simulink library "MOST_Lib"  (R2020b)
settings: Solver=VariableStepAuto  StartTime=0.0  StopTime=10.0  RelTol=1e-3
undefined symbols (not defined in the file): simu, wind, windTurbine, windturbine, X, Y, Z
libraries: nesl_utility x54, sm_lib x50, simulink x4, simulink_extras x1, pid_lib x1, WECSim_Lib_Body_Elements x1
(part 1 of 3)
settings Model: Creator=d060241  LastModifiedBy=akeeste
settings DebuggingCC: UnconnectedInputMsg=none  UnconnectedOutputMsg=none  UnconnectedLineMsg=none
settings ModelReferenceCC: EnableRefExpFcnMdlSchedulingChecks=off

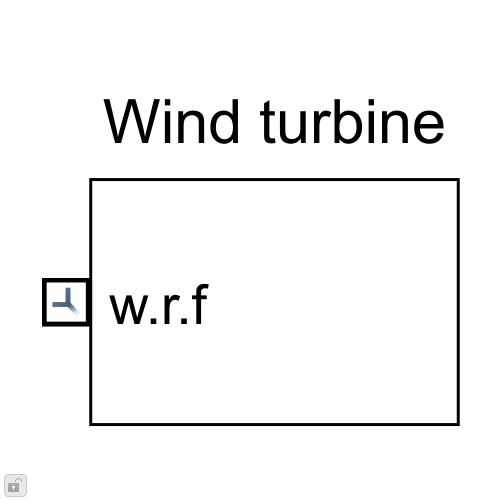
[thumbnail: Simulink's stored preview of the top-level diagram]
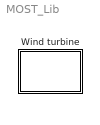
== system MOST_Lib ==
  Wind turbine : Subsystem  VariantControl=sv_1_IEA15MW  mask{windTurbine=windTurbine, BEMstruct=windTurbine.BEMstruct}
      mask prompts: windTurbine "Wind Number:"; BEMstruct "BEM structure"
      mask init:
      | %% Variand sybsystems
      | h = [gcb '/Aerodynamics + Control/Aeroloads/Look-up Tables'];
      | responseName = ['sv_t' num2str(windTurbine.number) '_AeroLoads0'];
      | set_param(h,'VariantControl',responseName);
      | 
      | h = [gcb '/Aerodynamics + Control/Aeroloads/BEM'];
      | responseName = ['sv_t' num2str(windTurbine.number) '_AeroLoads1'];
      | set_param(h,'VariantControl',responseName);
      | 
      | h = [gcb '/Aerodynamics + Control/Control/Baseline'];
      | responseName = ['sv_t' num2str(windTurbine.number) '_control0'];
      | set_param(h,'VariantControl',responseName);
      | 
      | h = [gcb '/Aerodynamics + Control/Control/ROSCO'];
      | responseName = ['sv_t' num2str(windTurbine.number) '_control1'];
      | set_param(h,'VariantControl',responseName);
      | 
      | %% Body properties
      | h1=[gcb '/Tower/Body Properties Tower'];
      | geomFile=windTurbine.geometryFileTower;
      | set_param(h1,'ExtGeomFileName',geomFile);
      | geomType='STEP';
      | 
      | h1=[gcb '/Nacelle/Body Properties Nacelle'];
      | geomFile=windTurbine.geometryFileNacelle;
      | set_param(h1,'ExtGeomFileName',geomFile);
      | geomType='STEP';
      | 
      | h1=[gcb '/Hub/Body Properties Hub'];
      | geomFile=windTurbine.geometryFileHub;
      | set_param(h1,'ExtGeomFileName',geomFile);
      | geomType='STEP';
      | 
      | h1=[gcb '/Blade 1/Blade/Body Properties Blade'];
      | geomFile=windTurbine.geometryFileBlade;
      | set_param(h1,'ExtGeomFileName',geomFile);
      | geomType='STEP';
      | 
      | h1=[gcb '/Blade 2/Blade/Body Properties Blade'];
      | geomFile=windTurbine.geometryFileBlade;
      | set_param(h1,'ExtGeomFileName',geomFile);
      | geomType='STEP';
      | 
      | h1=[gcb '/Blade 3/Blade/Body Properties Blade'];
      | geomFile=windTurbine.geometryFileBlade;
      | set_param(h1,'ExtGeomFileName',geomFile);
      | geomType='STEP';
      | 
      | 
      | %% toWorkSpace: outputs
      | h=[gcb '/Outputs/To Workspace'];
      | responseName=['windTurbine' num2str(windTurbine.number) '_out'];
      | set_param(h,'VariableName',responseName);
      | 
      | 
      | %% Goto
      | h=[gcb '/Nacelle/NacXdot'];
      | GotoName=['NacXdot' num2str(windTurbine.number)];
      | set_param(h,'GotoTag',GotoName);
      | 
      | h=[gcb '/Nacelle/NacelleAcceleration'];
      | GotoName=['NacAcc' num2str(windTurbine.number)];
      | set_param(h,'GotoTag',GotoName);
      | 
      | h=[gcb '/Blade 1/bladeRootLoad/blade1RootLoad'];
      | GotoName=['blade1RootLoad' num2str(windTurbine.number)];
      | set_param(h,'GotoTag',GotoName);
      | 
      | h=[gcb '/Blade 2/bladeRootLoad/blade2RootLoad'];
      | GotoName=['blade2RootLoad' num2str(windTurbine.number)];
      | set_param(h,'GotoTag',GotoName);
      | 
      | h=[gcb '/Blade 3/bladeRootLoad/blade3RootLoad'];
      | GotoName=['blade3RootLoad' num2str(windTurbine.number)];
      | set_param(h,'GotoTag',GotoName);
      | 
      | h=[gcb '/Aerodynamics + Control/Aeroloads/BEM/Hub wind speed/WindSpeed'];
      | GotoName=['WindSpeed' num2str(windTurbine.number)];
      | set_param(h,'GotoTag',GotoName);
      | 
      | h=[gcb '/Aerodynamics + Control/Aeroloads/Look-up Tables/Relative Wind/Hub wind speed/WindSpeed'];
      | GotoName=['WindSpeed' num2str(windTurbine.number)];
      | set_param(h,'GotoTag',GotoName);
      | 
      | h=[gcb '/TowerBaseLoad/TowerBaseLoad'];
      | GotoName=['TowerBaseLoad' num2str(windTurbine.number)];
      | set_param(h,'GotoTag',GotoName);
      | 
      | h=[gcb '/TowerTopLoad and deltaYaw/TowerTopLoad'];
      | GotoName=['TowerTopLoad' num2str(windTurbine.number)];
      | set_param(h,'GotoTag',GotoName);
      | 
      | h=[gcb '/TowerTopLoad and deltaYaw/deltaYaw'];
      | GotoName=['DeltaYaw' num2str(windTurbine.number)];
      | set_param(h,'GotoTag',GotoName);
      | 
      | h=[gcb '/Aerodynamics + Control/Goto_Power'];
      | GotoName=['TurbinePower' num2str(windTurbine.number)];
      | set_param(h,'GotoTag',GotoName);
      | 
      | h=[gcb '/Aerodynamics + Control/Goto_GenTorque'];
      | GotoName=['GenTorque' num2str(windTurbine.number)];
      | set_param(h,'GotoTag',GotoName);
      | 
      | h=[gcb '/Aerodynamics + Control/Goto_BladePitch'];
      | GotoName=['BladePitch' num2str(windTurbine.number)];
      | set_param(h,'GotoTag',GotoName);
      | 
      | h=[gcb '/Aerodynamics + Control/Goto_Azimuth'];
      | GotoName=['Azimuth' num2str(windTurbine.number)];
      | set_param(h,'GotoTag',GotoName);
      | 
      | h=[gcb '/Aerodynamics + Control/Goto_F_aero'];
      | GotoName=['F_aero' num2str(windTurbine.number)];
      | set_param(h,'GotoTag',GotoName);
      | 
      | h=[gcb '/Aerodynamics + Control/Goto_RotorSpeed'];
      | GotoName=['RotorSpeed' num2str(windTurbine.number)];
      | set_param(h,'GotoTag',GotoName);
      | 
      | 
      | 
      | %% From
      | h=[gcb '/Aerodynamics + Control/Yaw Control/WindSpeed'];
      | fromName=['WindSpeed' num2str(windTurbine.number)];
      | set_param(h,'GotoTag',fromName);
      | 
      | h=[gcb '/Aerodynamics + Control/Control/ROSCO/WindSpeed'];
      | fromName=['WindSpeed' num2str(windTurbine.number)];
      | set_param(h,'GotoTag',fromName);
      | 
      | h=[gcb '/Aerodynamics + Control/Control/ROSCO/NacXdot'];
      | fromName=['NacXdot' num2str(windTurbine.number)];
      | set_param(h,'GotoTag',fromName);
      | 
      | h=[gcb '/Outputs/WindSpeed'];
      | fromName=['WindSpeed' num2str(windTurbine.number)];
      | set_param(h,'GotoTag',fromName);
      | 
      | h=[gcb '/Outputs/TurbinePower'];
      | fromName=['TurbinePower' num2str(windTurbine.number)];
      | set_param(h,'GotoTag',fromName);
      | 
      | h=[gcb '/Outputs/RotorSpeed'];
      | fromName=['RotorSpeed' num2str(windTurbine.number)];
      | set_param(h,'GotoTag',fromName); 
      | 
      | h=[gcb '/Outputs/BladePitch'];
      | fromName=['BladePitch' num2str(windTurbine.number)];
      | set_param(h,'GotoTag',fromName);
      | 
      | h=[gcb '/Outputs/NacelleAcceleration'];
      | fromName=['NacAcc' num2str(windTurbine.number)];
      | set_param(h,'GotoTag',fromName);
      | 
      | h=[gcb '/Outputs/NacXdot'];
      | fromName=['NacXdot' num2str(windTurbine.number)];
      | set_param(h,'GotoTag',fromName);
      | 
      | h=[gcb '/Outputs/TowerBaseLoad'];
      | fromName=['TowerBaseLoad' num2str(windTurbine.number)];
      | set_param(h,'GotoTag',fromName);
      | 
      | h=[gcb '/Outputs/TowerTopLoad'];
      | fromName=['TowerTopLoad' num2str(windTurbine.number)];
      | set_param(h,'GotoTag',fromName);
      | 
      | h=[gcb '/Outputs/blade1RootLoad'];
      | fromName=['blade1RootLoad' num2str(windTurbine.number)];
      | set_param(h,'GotoTag',fromName);
      | 
      | h=[gcb '/Outputs/GenTorque'];
      | fromName=['GenTorque' num2str(windTurbine.number)];
      | set_param(h,'GotoTag',fromName);
      | 
      | h=[gcb '/Outputs/Azimuth'];
      | fromName=['Azimuth' num2str(windTurbine.number)];
      | set_param(h,'GotoTag',fromName);
      | 
      | h=[gcb '/Outputs/F_aero'];
      | fromName=['F_aero' num2str(windTurbine.number)];
      | set_param(h,'GotoTag',fromName);
      | 
      | h=[gcb '/Outputs/deltaYaw'];
      | fromName=['DeltaYaw' num2str(windTurbine.number)];
      | set_param(h,'GotoTag',fromName);
      | 
      | h=[gcb '/Outputs/blade2RootLoad'];
      | fromName=['blade2RootLoad' num2str(windTurbine.number)];
      | set_param(h,'GotoTag',fromName);
      | 
      | h=[gcb '/Outputs/blade3RootLoad'];
      | fromName=['blade3RootLoad' num2str(windTurbine.number)];
      | set_param(h,'GotoTag',fromName);
      mask Display: image('$imagefile');

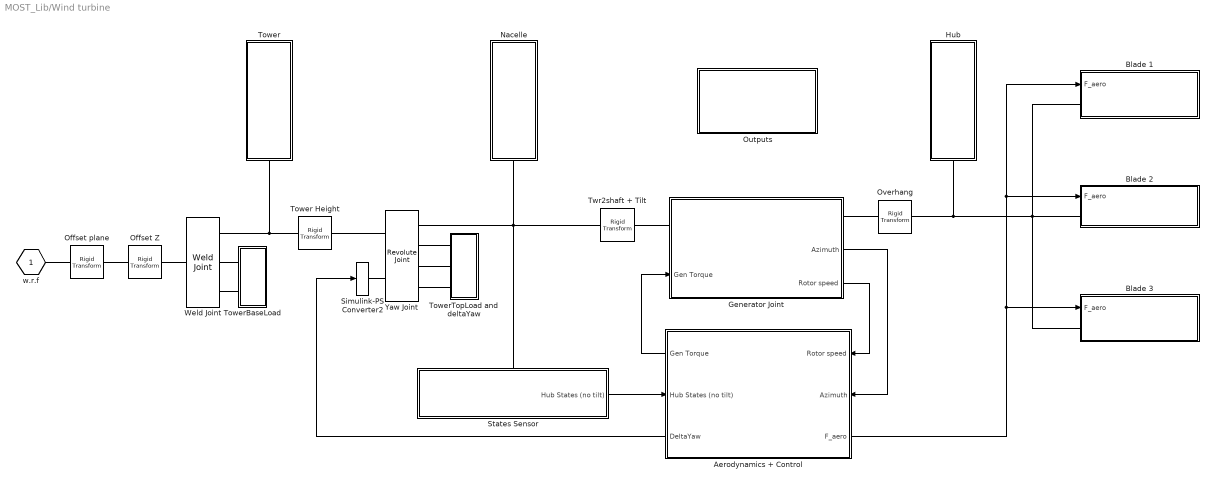
== system MOST_Lib/Wind turbine ==
  Aerodynamics + Control : Subsystem  VariantControl=sv_control2
      settings: PortSchema="{\"entries\":[{\"content\":{\"sides\":[{\"content\":{\"connectorIds\":[\"In1\",\"In2\",\"Out3\"]},\"type\":\"ConnectorPlacement.EquallySpacedRectSide\",\"uuid\":\"f605537b-ff67-4139-9e35-b0b4424af1fd\"},{\"content\":{\"connectorIds\":[\"Out1\",\"In3\",\"Out2\"],\"side\":\"RIGHT\"},\"type\":\"ConnectorPlacement.EquallySpacedRectSide\",\"uuid\":\"3a18d562-2e9f-426a-bf17-957f05b26031\"},{\"content\":{\"side\":\"TOP\"},\"type\":\"ConnectorPlacement.EquallySpacedRectSide\",\"uuid\":\"40c82717-587d-4d52-9cee-a57347508196\"}]},\"type\":\"ConnectorPlacement.EquallySpacedConnector\",\"uuid\":\"179eafe9-7dd0-4a47-b537-f46cd85fd5cb\"}],\"packageUris\":[\"http://schema.mathworks.com/mf0/Connector/R2020b\"],\"version\":\"1.0\"}"
  Blade 1 : Subsystem
  Blade 2 : Subsystem
  Blade 3 : Subsystem
  Generator Joint : Subsystem
      settings: PortSchema="{\"entries\":[{\"content\":{\"sides\":[{\"content\":{\"connectorIds\":[\"LConn1\",\"In1\"]},\"type\":\"ConnectorPlacement.EquallySpacedRectSide\",\"uuid\":\"aa43b6bb-07e6-4639-8984-05e2f05037c7\"},{\"content\":{\"connectorIds\":[\"RConn1\",\"Out1\",\"Out2\"],\"side\":\"RIGHT\"},\"type\":\"ConnectorPlacement.EquallySpacedRectSide\",\"uuid\":\"5555dcdf-e304-4e73-b091-ea9b223dd22e\"},{\"content\":{\"side\":\"TOP\"},\"type\":\"ConnectorPlacement.EquallySpacedRectSide\",\"uuid\":\"9954d7ec-e15d-4078-b1e6-3c644a0ef755\"}]},\"type\":\"ConnectorPlacement.EquallySpacedConnector\",\"uuid\":\"b5c1905d-1ccd-4f5d-98bc-367249db9bf9\"}],\"packageUris\":[\"http://schema.mathworks.com/mf0/Connector/R2020b\"],\"version\":\"1.0\"}"
  Hub : Subsystem
  Nacelle : Subsystem
  Offset Z : sm_lib/Frames and Transforms/Rigid Transform  RotationMethod=None  FollAlignAxisA=+X  BaseAlignAxisA=+Y  FollAlignAxisB=+Y  BaseAlignAxisB=+Z  RotationStandardAxis=+Z  RotationAngle=0.0  RotationAngleUnits=deg  RotationArbitraryAxis=[0 0 1]  RotationSequenceAxes=FollowerAxes  RotationSequence=XYX  RotationSequenceAngles=[0 0 0]  RotationSequenceAnglesUnits=deg  RotationMatrix=[1 0 0; 0 1 0; 0 0 1]  Quaternion=[1 0 0 0]  TranslationMethod=StandardAxis  TranslationCartesianOffset=[0 0 0]  TranslationCartesianOffsetUnits=m  TranslationStandardAxis=+Z  TranslationStandardOffset=windTurbine.tower.offset  TranslationStandardOffsetUnits=m  TranslationROffset=0  TranslationROffsetUnits=m  TranslationThetaOffset=0  TranslationThetaOffsetUnits=deg  TranslationZOffset=0  TranslationZOffsetUnits=m
  Offset plane : sm_lib/Frames and Transforms/Rigid Transform  RotationMethod=None  FollAlignAxisA=+X  BaseAlignAxisA=+Y  FollAlignAxisB=+Y  BaseAlignAxisB=+Z  RotationStandardAxis=+Z  RotationAngle=0.0  RotationAngleUnits=deg  RotationArbitraryAxis=[0 0 1]  RotationSequenceAxes=FollowerAxes  RotationSequence=XYX  RotationSequenceAngles=[0 0 0]  RotationSequenceAnglesUnits=deg  RotationMatrix=[1 0 0; 0 1 0; 0 0 1]  Quaternion=[1 0 0 0]  TranslationMethod=Cartesian  TranslationCartesianOffset=[windTurbine.offset_plane 0]  TranslationCartesianOffsetUnits=m  TranslationStandardAxis=+Z  TranslationStandardOffset=[windTurbine.offset_plane 0]  TranslationStandardOffsetUnits=m  TranslationROffset=0  TranslationROffsetUnits=m  TranslationThetaOffset=0  TranslationThetaOffsetUnits=deg  TranslationZOffset=0  TranslationZOffsetUnits=m
  Outputs : Subsystem
  Overhang : sm_lib/Frames and Transforms/Rigid Transform  RotationMethod=None  FollAlignAxisA=+X  BaseAlignAxisA=+Y  FollAlignAxisB=+Y  BaseAlignAxisB=+Z  RotationStandardAxis=+Z  RotationAngle=0.0  RotationAngleUnits=deg  RotationArbitraryAxis=[0 0 1]  RotationSequenceAxes=FollowerAxes  RotationSequence=XYX  RotationSequenceAngles=[0 0 0]  RotationSequenceAnglesUnits=deg  RotationMatrix=[1 0 0; 0 1 0; 0 0 1]  Quaternion=[1 0 0 0]  TranslationMethod=StandardAxis  TranslationCartesianOffset=[0 0 0]  TranslationCartesianOffsetUnits=m  TranslationStandardAxis=+X  TranslationStandardOffset=windTurbine.hub.overhang  TranslationStandardOffsetUnits=m  TranslationROffset=0  TranslationROffsetUnits=m  TranslationThetaOffset=0  TranslationThetaOffsetUnits=deg  TranslationZOffset=0  TranslationZOffsetUnits=m
  Simulink-PS Converter2 : nesl_utility/Simulink-PS Converter  PhysicalDomain=network_engine_domain  SubClassName=ps_input  LeftPortType=input  RightPortType=output  PseudoPeriodic=off  Frequencies=[]  NoiseDistribution=none  NoiseParameters=[]  Unit=rad  AffineConversion=off  FilteringAndDerivatives=filter  SimscapeFilterOrder=2  InputFilterTimeConstant=0.1  UdotUserProvided=0
  States Sensor : Subsystem
      settings: PortSchema="{\"entries\":[{\"content\":{\"sides\":[{\"content\":{\"connectorIds\":[\"LConn1\"]},\"type\":\"ConnectorPlacement.EquallySpacedRectSide\",\"uuid\":\"e2551c45-43da-4d17-b6e7-45dc7a2744e2\"},{\"content\":{\"side\":\"RIGHT\"},\"type\":\"ConnectorPlacement.EquallySpacedRectSide\",\"uuid\":\"3e623cb2-59ea-443e-940e-3b000cef6b1c\"},{\"content\":{\"side\":\"TOP\"},\"type\":\"ConnectorPlacement.EquallySpacedRectSide\",\"uuid\":\"fecc8c6a-e08d-489d-84d9-b9b5d67a9881\"},{\"content\":{\"connectorIds\":[\"Out1\"],\"side\":\"BOTTOM\"},\"type\":\"ConnectorPlacement.EquallySpacedRectSide\",\"uuid\":\"df37bb48-66b2-4e60-9226-2f9bc134eb2e\"}]},\"type\":\"ConnectorPlacement.EquallySpacedConnector\",\"uuid\":\"7584ff8d-439c-42ba-a06a-3f3add1a835d\"}],\"packageUris\":[\"http://schema.mathworks.com/mf0/Connector/R2020b\"],\"version\":\"1.0\"}"
  Tower : Subsystem
  Tower Height : sm_lib/Frames and Transforms/Rigid Transform  RotationMethod=None  FollAlignAxisA=+X  BaseAlignAxisA=+Y  FollAlignAxisB=+Y  BaseAlignAxisB=+Z  RotationStandardAxis=+Z  RotationAngle=0.0  RotationAngleUnits=deg  RotationArbitraryAxis=[0 0 1]  RotationSequenceAxes=FollowerAxes  RotationSequence=XYX  RotationSequenceAngles=[0 0 0]  RotationSequenceAnglesUnits=deg  RotationMatrix=[1 0 0; 0 1 0; 0 0 1]  Quaternion=[1 0 0 0]  TranslationMethod=StandardAxis  TranslationCartesianOffset=[0 0 0]  TranslationCartesianOffsetUnits=m  TranslationStandardAxis=+Z  TranslationStandardOffset=windTurbine.tower.height  TranslationStandardOffsetUnits=m  TranslationROffset=0  TranslationROffsetUnits=m  TranslationThetaOffset=0  TranslationThetaOffsetUnits=deg  TranslationZOffset=0  TranslationZOffsetUnits=m
  TowerBaseLoad : Subsystem
  TowerTopLoad and deltaYaw : Subsystem
  "Twr2shaft + Tilt " : sm_lib/Frames and Transforms/Rigid Transform  RotationMethod=StandardAxis  FollAlignAxisA=+X  BaseAlignAxisA=+Y  FollAlignAxisB=+Y  BaseAlignAxisB=+Z  RotationStandardAxis=+Y  RotationAngle=windTurbine.nacelle.tiltangle  RotationAngleUnits=deg  RotationArbitraryAxis=[0 0 1]  RotationSequenceAxes=FollowerAxes  RotationSequence=XYX  RotationSequenceAngles=[0 0 0]  RotationSequenceAnglesUnits=deg  RotationMatrix=[1 0 0; 0 1 0; 0 0 1]  Quaternion=[1 0 0 0]  TranslationMethod=StandardAxis  TranslationCartesianOffset=[0 0 0]  TranslationCartesianOffsetUnits=m  TranslationStandardAxis=+Z  TranslationStandardOffset=windTurbine.nacelle.Twr2Shft  TranslationStandardOffsetUnits=m  TranslationROffset=0  TranslationROffsetUnits=m  TranslationThetaOffset=0  TranslationThetaOffsetUnits=deg  TranslationZOffset=0  TranslationZOffsetUnits=m
  Weld Joint : sm_lib/Joints/Weld Joint  JointMode=Normal  CompositeWrenchDir=FollowerOnBase  CompositeWrenchFrame=BaseFrame  SenseConstraintForce=on  SenseConstraintTorque=on  SenseTotalForce=off  SenseTotalTorque=off
  Yaw Joint : sm_lib/Joints/Revolute Joint  JointMode=Normal  CompositeWrenchDir=FollowerOnBase  CompositeWrenchFrame=BaseFrame  SenseConstraintForce=off  SenseConstraintTorque=off  SenseTotalForce=on  SenseTotalTorque=on  PositionTargetSpecify=on  PositionTargetPriority=Low  PositionTargetValue=0  PositionTargetValueUnits=deg  VelocityTargetSpecify=on  VelocityTargetPriority=Low  VelocityTargetValue=0  VelocityTargetValueUnits=deg/s  EquilibriumPosition=0  EquilibriumPositionUnits=deg  SpringStiffness=0.000001  SpringStiffnessUnits=N*m/deg  DampingCoefficient=0.000001  DampingCoefficientUnits=N*m/(deg/s)  LowerLimitSpecify=off  LowerLimitBound=-90  LowerLimitBoundUnits=deg  LowerLimitStiffness=1e4  LowerLimitStiffnessUnits=N*m/deg  LowerLimitDamping=10  LowerLimitDampingUnits=N*m/(deg/s)  LowerLimitTransitionRegionWidth=0.1  LowerLimitTransitionRegionWidthUnits=deg  UpperLimitSpecify=off  UpperLimitBound=90  UpperLimitBoundUnits=deg  UpperLimitStiffness=1e4  UpperLimitStiffnessUnits=N*m/deg  UpperLimitDamping=10  UpperLimitDampingUnits=N*m/(deg/s)  UpperLimitTransitionRegionWidth=0.1  UpperLimitTransitionRegionWidthUnits=deg  TorqueActuationMode=ComputedTorque  MotionActuationMode=InputMotion  SensePosition=on  SenseVelocity=off  SenseAcceleration=off  SenseTorqueForce=off  SenseLowerLimitTorqueForce=off  SenseUpperLimitTorqueForce=off
  w.r.f : PMIOPort  Side=Right
  wires:
  Aerodynamics + Control/3(F_aero) -> Blade 1/1(F_aero), Blade 2/1(F_aero), Blade 3/1(F_aero)
  Aerodynamics + Control/2(DeltaYaw) -> Simulink-PS Converter2/1
  States Sensor/1(Hub States (no tilt)) -> Aerodynamics + Control/3(Hub States (no tilt))
  Aerodynamics + Control/1(Gen Torque) -> Generator Joint/1(Gen Torque)
  Generator Joint/1(Azimuth) -> Aerodynamics + Control/2(Azimuth)
  Generator Joint/2(" Rotor speed") -> Aerodynamics + Control/1(" Rotor speed")
  connections:
  Nacelle/LConn1 -- States Sensor/LConn1 -- Yaw Joint/RConn1 -- "Twr2shaft + Tilt "/LConn1
  Tower/LConn1 -- Weld Joint/RConn1 -- Tower Height/LConn1
  Tower Height/RConn1 -- Yaw Joint/LConn1
  Offset plane/RConn1 -- Offset Z/LConn1
  Offset Z/RConn1 -- Weld Joint/LConn1
  Overhang/RConn1 -- Hub/LConn1 -- Blade 1/LConn1 -- Blade 2/LConn1 -- Blade 3/LConn1
  Weld Joint/RConn2 -- TowerBaseLoad/LConn1
  Weld Joint/RConn3 -- TowerBaseLoad/LConn2
  Yaw Joint/RConn2 -- TowerTopLoad and deltaYaw/LConn1
  Offset plane/LConn1 -- w.r.f/RConn1
  Yaw Joint/RConn3 -- TowerTopLoad and deltaYaw/LConn2
  Yaw Joint/RConn4 -- TowerTopLoad and deltaYaw/LConn3
  Simulink-PS Converter2/RConn1 -- Yaw Joint/LConn2
  Generator Joint/LConn1 -- "Twr2shaft + Tilt "/RConn1
  Generator Joint/RConn1 -- Overhang/LConn1

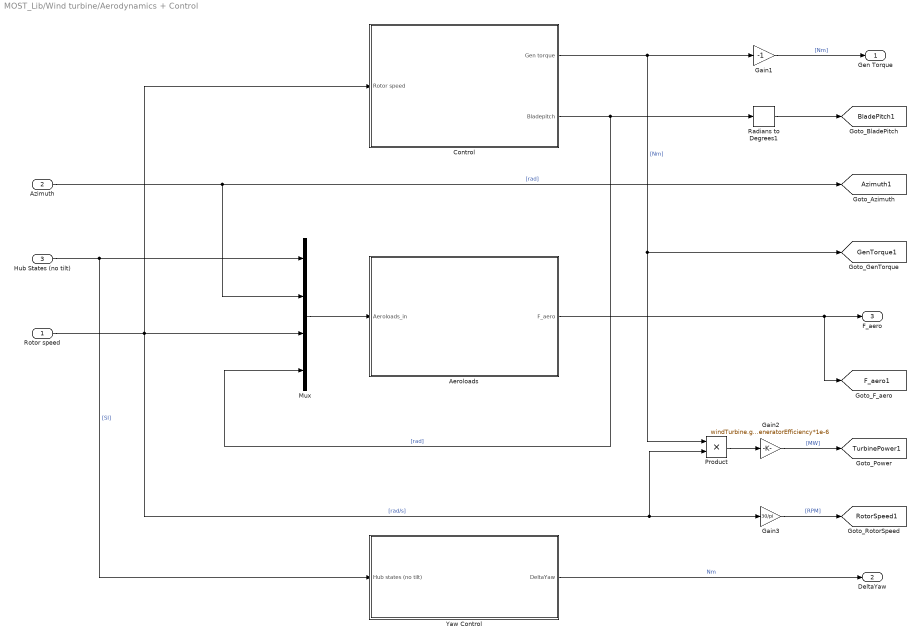
== system MOST_Lib/Wind turbine/Aerodynamics + Control ==
  " Rotor speed" : Inport
  Azimuth : Inport  Port=2
  Hub States (no tilt) : Inport  Port=3
  Aeroloads : Subsystem  Variant=on  AllowZeroVariantControls=on
  Control : Subsystem  Variant=on  VariantControl=sv_IEA10MW  AllowZeroVariantControls=on
  Gain1 : Gain  Gain=-1
  Gain2 : Gain  Gain=windTurbine.generatorEfficiency*1e-6
  Gain3 : Gain  Gain=30/pi
  Mux : Mux
  Product : Product
  Radians to Degrees1 : simulink_extras/Transformations/Radians to Degrees
  Yaw Control : Subsystem
  Gen Torque : Outport  VectorParamsAs1DForOutWhenUnconnected=off
  DeltaYaw : Outport  Port=2
  F_aero : Outport  Port=3
  tag scope: Azimuth1=global, BladePitch1=global, F_aero1=global, GenTorque1=global, RotorSpeed1=global, TurbinePower1=global
  wires:
  Control/2(Bladepitch) -> Mux/4, Radians to Degrees1/1  "[rad]"
  Control/1(Gen torque) -> Product/1, [GenTorque1], Gain1/1  "[Nm]"
  Product/1 -> Gain2/1
  Azimuth/1 -> Mux/2, [Azimuth1]  "[rad]"
  Gain3/1 -> [RotorSpeed1]  "[RPM]"
  Gain1/1 -> Gen Torque/1  "[Nm]"
  Gain2/1 -> [TurbinePower1]  "[MW]"
  Radians to Degrees1/1 -> [BladePitch1]
  Hub States (no tilt)/1 -> Yaw Control/1(Hub states (no tilt)), Mux/1  "[SI]"
  Mux/1 -> Aeroloads/1(Aeroloads_in)
  " Rotor speed"/1 -> Control/1(Rotor speed), Product/2, Gain3/1, Mux/3  "[rad/s]"
  Aeroloads/1(F_aero) -> F_aero/1, [F_aero1]
  Yaw Control/1(DeltaYaw) -> DeltaYaw/1  "Nm"

== system MOST_Lib/Wind turbine/Blade 1 ==
  F_aero : Inport
  Blade : Subsystem
  Demux : Demux  Outputs=6
  Precone : sm_lib/Frames and Transforms/Rigid Transform  RotationMethod=StandardAxis  FollAlignAxisA=+X  BaseAlignAxisA=+Y  FollAlignAxisB=+Y  BaseAlignAxisB=+Z  RotationStandardAxis=-Y  RotationAngle=windTurbine.hub.precone  RotationAngleUnits=deg  RotationArbitraryAxis=[0 0 1]  RotationSequenceAxes=FollowerAxes  RotationSequence=XYX  RotationSequenceAngles=[0 0 0]  RotationSequenceAnglesUnits=deg  RotationMatrix=[1 0 0; 0 1 0; 0 0 1]  Quaternion=[1 0 0 0]  TranslationMethod=None  TranslationCartesianOffset=[0 0 0]  TranslationCartesianOffsetUnits=m  TranslationStandardAxis=+Z  TranslationStandardOffset=0  TranslationStandardOffsetUnits=m  TranslationROffset=0  TranslationROffsetUnits=m  TranslationThetaOffset=0  TranslationThetaOffsetUnits=deg  TranslationZOffset=0  TranslationZOffsetUnits=m
  Rhub : sm_lib/Frames and Transforms/Rigid Transform  RotationMethod=None  FollAlignAxisA=+X  BaseAlignAxisA=+Y  FollAlignAxisB=+Y  BaseAlignAxisB=+Z  RotationStandardAxis=+Z  RotationAngle=0.0  RotationAngleUnits=deg  RotationArbitraryAxis=[0 0 1]  RotationSequenceAxes=FollowerAxes  RotationSequence=XYX  RotationSequenceAngles=[0 0 0]  RotationSequenceAnglesUnits=deg  RotationMatrix=[1 0 0; 0 1 0; 0 0 1]  Quaternion=[1 0 0 0]  TranslationMethod=StandardAxis  TranslationCartesianOffset=[0 0 0]  TranslationCartesianOffsetUnits=m  TranslationStandardAxis=+Z  TranslationStandardOffset=windTurbine.hub.Rhub  TranslationStandardOffsetUnits=m  TranslationROffset=0  TranslationROffsetUnits=m  TranslationThetaOffset=0  TranslationThetaOffsetUnits=deg  TranslationZOffset=0  TranslationZOffsetUnits=m
  Selector : Selector  NumberOfDimensions=2  InputPortWidth=3  IndexOptions=Select all,Index vector (dialog)  Indices=[1 3],1  OutputSizes=1,1
  Simulink-PS Converter{,1..5} (6 alike) : nesl_utility/Simulink-PS Converter  PhysicalDomain=network_engine_domain  SubClassName=ps_input  LeftPortType=input  RightPortType=output  PseudoPeriodic=off  Frequencies=[]  NoiseDistribution=none  NoiseParameters=[]  Unit=1  AffineConversion=off  FilteringAndDerivatives=provide  SimscapeFilterOrder=1  InputFilterTimeConstant=0.001  UdotUserProvided=0
  Weld Joint : sm_lib/Joints/Weld Joint  JointMode=Normal  CompositeWrenchDir=FollowerOnBase  CompositeWrenchFrame=BaseFrame  SenseConstraintForce=on  SenseConstraintTorque=on  SenseTotalForce=off  SenseTotalTorque=off
  aerodynamic forces : sm_lib/Forces and Torques/External Force and Torque  EnableForceX=on  EnableForceY=on  EnableForceZ=on  EnableForce=off  ForceResolutionFrame=AttachedFrame  EnableTorqueX=on  EnableTorqueY=on  EnableTorqueZ=on  EnableTorque=off  TorqueResolutionFrame=AttachedFrame
  bladeRootLoad : Subsystem
  Blade1 Root : PMIOPort  Side=Left
  wires:
  Demux/5 -> Simulink-PS Converter4/1
  Demux/3 -> Simulink-PS Converter2/1
  Demux/4 -> Simulink-PS Converter3/1
  Demux/6 -> Simulink-PS Converter5/1
  Demux/1 -> Simulink-PS Converter/1
  F_aero/1 -> Selector/1
  Selector/1 -> Demux/1
  Demux/2 -> Simulink-PS Converter1/1
  connections:
  Rhub/LConn1 -- Precone/RConn1
  Rhub/RConn1 -- Weld Joint/LConn1
  Blade1 Root/RConn1 -- Precone/LConn1
  Weld Joint/RConn1 -- aerodynamic forces/RConn1 -- Blade/LConn1
  Simulink-PS Converter4/RConn1 -- aerodynamic forces/LConn5
  Simulink-PS Converter1/RConn1 -- aerodynamic forces/LConn2
  Simulink-PS Converter5/RConn1 -- aerodynamic forces/LConn6
  aerodynamic forces/LConn4 -- Simulink-PS Converter3/RConn1
  Simulink-PS Converter/RConn1 -- aerodynamic forces/LConn1
  Simulink-PS Converter2/RConn1 -- aerodynamic forces/LConn3
  Weld Joint/RConn2 -- bladeRootLoad/LConn1
  Weld Joint/RConn3 -- bladeRootLoad/LConn2

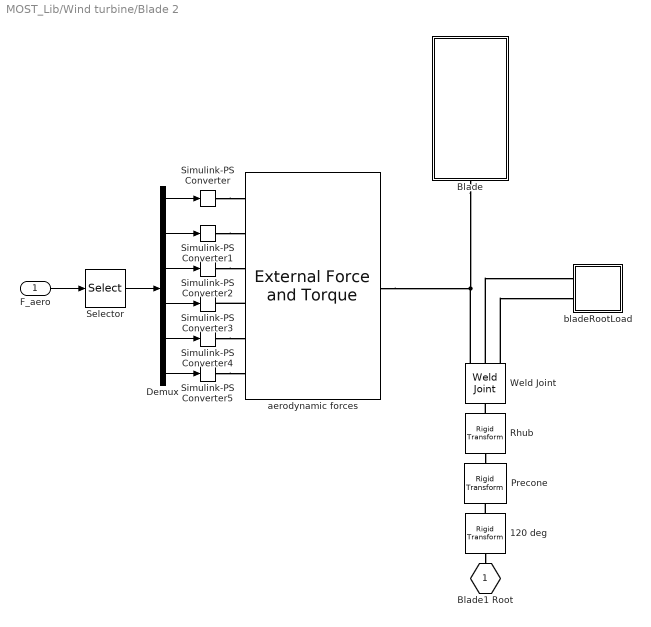
== system MOST_Lib/Wind turbine/Blade 2 ==
  F_aero : Inport
  120 deg : sm_lib/Frames and Transforms/Rigid Transform  RotationMethod=StandardAxis  FollAlignAxisA=+X  BaseAlignAxisA=+Y  FollAlignAxisB=+Y  BaseAlignAxisB=+Z  RotationStandardAxis=+X  RotationAngle=120  RotationAngleUnits=deg  RotationArbitraryAxis=[0 0 1]  RotationSequenceAxes=FollowerAxes  RotationSequence=XYX  RotationSequenceAngles=[0 0 0]  RotationSequenceAnglesUnits=deg  RotationMatrix=[1 0 0; 0 1 0; 0 0 1]  Quaternion=[1 0 0 0]  TranslationMethod=None  TranslationCartesianOffset=[0 0 0]  TranslationCartesianOffsetUnits=m  TranslationStandardAxis=+Z  TranslationStandardOffset=0  TranslationStandardOffsetUnits=m  TranslationROffset=0  TranslationROffsetUnits=m  TranslationThetaOffset=0  TranslationThetaOffsetUnits=deg  TranslationZOffset=0  TranslationZOffsetUnits=m
  Blade : Subsystem
  Demux : Demux  Outputs=6
  Precone : sm_lib/Frames and Transforms/Rigid Transform  RotationMethod=StandardAxis  FollAlignAxisA=+X  BaseAlignAxisA=+Y  FollAlignAxisB=+Y  BaseAlignAxisB=+Z  RotationStandardAxis=-Y  RotationAngle=windTurbine.hub.precone  RotationAngleUnits=deg  RotationArbitraryAxis=[0 0 1]  RotationSequenceAxes=FollowerAxes  RotationSequence=XYX  RotationSequenceAngles=[0 0 0]  RotationSequenceAnglesUnits=deg  RotationMatrix=[1 0 0; 0 1 0; 0 0 1]  Quaternion=[1 0 0 0]  TranslationMethod=None  TranslationCartesianOffset=[0 0 0]  TranslationCartesianOffsetUnits=m  TranslationStandardAxis=+Z  TranslationStandardOffset=0  TranslationStandardOffsetUnits=m  TranslationROffset=0  TranslationROffsetUnits=m  TranslationThetaOffset=0  TranslationThetaOffsetUnits=deg  TranslationZOffset=0  TranslationZOffsetUnits=m
  Rhub : sm_lib/Frames and Transforms/Rigid Transform  RotationMethod=None  FollAlignAxisA=+X  BaseAlignAxisA=+Y  FollAlignAxisB=+Y  BaseAlignAxisB=+Z  RotationStandardAxis=+Z  RotationAngle=0.0  RotationAngleUnits=deg  RotationArbitraryAxis=[0 0 1]  RotationSequenceAxes=FollowerAxes  RotationSequence=XYX  RotationSequenceAngles=[0 0 0]  RotationSequenceAnglesUnits=deg  RotationMatrix=[1 0 0; 0 1 0; 0 0 1]  Quaternion=[1 0 0 0]  TranslationMethod=StandardAxis  TranslationCartesianOffset=[0 0 0]  TranslationCartesianOffsetUnits=m  TranslationStandardAxis=+Z  TranslationStandardOffset=windTurbine.hub.Rhub  TranslationStandardOffsetUnits=m  TranslationROffset=0  TranslationROffsetUnits=m  TranslationThetaOffset=0  TranslationThetaOffsetUnits=deg  TranslationZOffset=0  TranslationZOffsetUnits=m
  Selector : Selector  NumberOfDimensions=2  InputPortWidth=3  IndexOptions=Select all,Index vector (dialog)  Indices=[1 3],2  OutputSizes=1,1
  Simulink-PS Converter{,1..5} (6 alike) : nesl_utility/Simulink-PS Converter  PhysicalDomain=network_engine_domain  SubClassName=ps_input  LeftPortType=input  RightPortType=output  PseudoPeriodic=off  Frequencies=[]  NoiseDistribution=none  NoiseParameters=[]  Unit=1  AffineConversion=off  FilteringAndDerivatives=provide  SimscapeFilterOrder=1  InputFilterTimeConstant=0.001  UdotUserProvided=0
  Weld Joint : sm_lib/Joints/Weld Joint  JointMode=Normal  CompositeWrenchDir=FollowerOnBase  CompositeWrenchFrame=BaseFrame  SenseConstraintForce=on  SenseConstraintTorque=on  SenseTotalForce=off  SenseTotalTorque=off
  aerodynamic forces : sm_lib/Forces and Torques/External Force and Torque  EnableForceX=on  EnableForceY=on  EnableForceZ=on  EnableForce=off  ForceResolutionFrame=AttachedFrame  EnableTorqueX=on  EnableTorqueY=on  EnableTorqueZ=on  EnableTorque=off  TorqueResolutionFrame=AttachedFrame
  bladeRootLoad : Subsystem
  Blade1 Root : PMIOPort  Side=Left
  wires:
  Demux/2 -> Simulink-PS Converter1/1
  Selector/1 -> Demux/1
  F_aero/1 -> Selector/1
  Demux/1 -> Simulink-PS Converter/1
  Demux/6 -> Simulink-PS Converter5/1
  Demux/4 -> Simulink-PS Converter3/1
  Demux/3 -> Simulink-PS Converter2/1
  Demux/5 -> Simulink-PS Converter4/1
  connections:
  Weld Joint/RConn3 -- bladeRootLoad/LConn2
  Weld Joint/RConn2 -- bladeRootLoad/LConn1
  Simulink-PS Converter2/RConn1 -- aerodynamic forces/LConn3
  Simulink-PS Converter/RConn1 -- aerodynamic forces/LConn1
  aerodynamic forces/LConn4 -- Simulink-PS Converter3/RConn1
  Simulink-PS Converter5/RConn1 -- aerodynamic forces/LConn6
  Simulink-PS Converter1/RConn1 -- aerodynamic forces/LConn2
  Simulink-PS Converter4/RConn1 -- aerodynamic forces/LConn5
  Blade/LConn1 -- aerodynamic forces/RConn1 -- Weld Joint/RConn1
  120 deg/RConn1 -- Precone/LConn1
  Rhub/RConn1 -- Weld Joint/LConn1
  Rhub/LConn1 -- Precone/RConn1
  120 deg/LConn1 -- Blade1 Root/RConn1

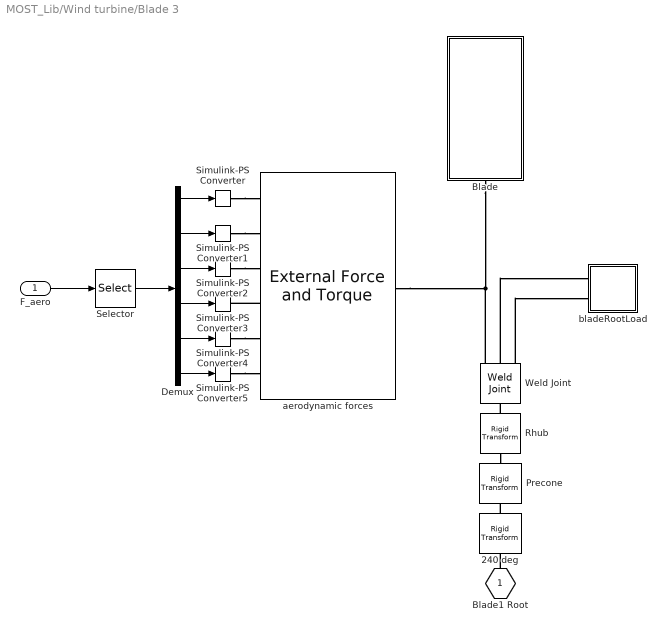
== system MOST_Lib/Wind turbine/Blade 3 ==
  F_aero : Inport
  240 deg : sm_lib/Frames and Transforms/Rigid Transform  RotationMethod=StandardAxis  FollAlignAxisA=+X  BaseAlignAxisA=+Y  FollAlignAxisB=+Y  BaseAlignAxisB=+Z  RotationStandardAxis=+X  RotationAngle=240  RotationAngleUnits=deg  RotationArbitraryAxis=[0 0 1]  RotationSequenceAxes=FollowerAxes  RotationSequence=XYX  RotationSequenceAngles=[0 0 0]  RotationSequenceAnglesUnits=deg  RotationMatrix=[1 0 0; 0 1 0; 0 0 1]  Quaternion=[1 0 0 0]  TranslationMethod=None  TranslationCartesianOffset=[0 0 0]  TranslationCartesianOffsetUnits=m  TranslationStandardAxis=+Z  TranslationStandardOffset=0  TranslationStandardOffsetUnits=m  TranslationROffset=0  TranslationROffsetUnits=m  TranslationThetaOffset=0  TranslationThetaOffsetUnits=deg  TranslationZOffset=0  TranslationZOffsetUnits=m
  Blade : Subsystem
  Demux : Demux  Outputs=6
  Precone : sm_lib/Frames and Transforms/Rigid Transform  RotationMethod=StandardAxis  FollAlignAxisA=+X  BaseAlignAxisA=+Y  FollAlignAxisB=+Y  BaseAlignAxisB=+Z  RotationStandardAxis=-Y  RotationAngle=windTurbine.hub.precone  RotationAngleUnits=deg  RotationArbitraryAxis=[0 0 1]  RotationSequenceAxes=FollowerAxes  RotationSequence=XYX  RotationSequenceAngles=[0 0 0]  RotationSequenceAnglesUnits=deg  RotationMatrix=[1 0 0; 0 1 0; 0 0 1]  Quaternion=[1 0 0 0]  TranslationMethod=None  TranslationCartesianOffset=[0 0 0]  TranslationCartesianOffsetUnits=m  TranslationStandardAxis=+Z  TranslationStandardOffset=0  TranslationStandardOffsetUnits=m  TranslationROffset=0  TranslationROffsetUnits=m  TranslationThetaOffset=0  TranslationThetaOffsetUnits=deg  TranslationZOffset=0  TranslationZOffsetUnits=m
  Rhub : sm_lib/Frames and Transforms/Rigid Transform  RotationMethod=None  FollAlignAxisA=+X  BaseAlignAxisA=+Y  FollAlignAxisB=+Y  BaseAlignAxisB=+Z  RotationStandardAxis=+Z  RotationAngle=0.0  RotationAngleUnits=deg  RotationArbitraryAxis=[0 0 1]  RotationSequenceAxes=FollowerAxes  RotationSequence=XYX  RotationSequenceAngles=[0 0 0]  RotationSequenceAnglesUnits=deg  RotationMatrix=[1 0 0; 0 1 0; 0 0 1]  Quaternion=[1 0 0 0]  TranslationMethod=StandardAxis  TranslationCartesianOffset=[0 0 0]  TranslationCartesianOffsetUnits=m  TranslationStandardAxis=+Z  TranslationStandardOffset=windTurbine.hub.Rhub  TranslationStandardOffsetUnits=m  TranslationROffset=0  TranslationROffsetUnits=m  TranslationThetaOffset=0  TranslationThetaOffsetUnits=deg  TranslationZOffset=0  TranslationZOffsetUnits=m
  Selector : Selector  NumberOfDimensions=2  InputPortWidth=3  IndexOptions=Select all,Index vector (dialog)  Indices=[1 3],3  OutputSizes=1,1
  Simulink-PS Converter{,1..5} (6 alike) : nesl_utility/Simulink-PS Converter  PhysicalDomain=network_engine_domain  SubClassName=ps_input  LeftPortType=input  RightPortType=output  PseudoPeriodic=off  Frequencies=[]  NoiseDistribution=none  NoiseParameters=[]  Unit=1  AffineConversion=off  FilteringAndDerivatives=provide  SimscapeFilterOrder=1  InputFilterTimeConstant=0.001  UdotUserProvided=0
  Weld Joint : sm_lib/Joints/Weld Joint  JointMode=Normal  CompositeWrenchDir=FollowerOnBase  CompositeWrenchFrame=BaseFrame  SenseConstraintForce=on  SenseConstraintTorque=on  SenseTotalForce=off  SenseTotalTorque=off
  aerodynamic forces : sm_lib/Forces and Torques/External Force and Torque  EnableForceX=on  EnableForceY=on  EnableForceZ=on  EnableForce=off  ForceResolutionFrame=AttachedFrame  EnableTorqueX=on  EnableTorqueY=on  EnableTorqueZ=on  EnableTorque=off  TorqueResolutionFrame=AttachedFrame
  bladeRootLoad : Subsystem
  Blade1 Root : PMIOPort  Side=Left
  wires:
  Demux/2 -> Simulink-PS Converter1/1
  Selector/1 -> Demux/1
  F_aero/1 -> Selector/1
  Demux/1 -> Simulink-PS Converter/1
  Demux/6 -> Simulink-PS Converter5/1
  Demux/4 -> Simulink-PS Converter3/1
  Demux/3 -> Simulink-PS Converter2/1
  Demux/5 -> Simulink-PS Converter4/1
  connections:
  Weld Joint/RConn3 -- bladeRootLoad/LConn2
  Weld Joint/RConn2 -- bladeRootLoad/LConn1
  Simulink-PS Converter2/RConn1 -- aerodynamic forces/LConn3
  Simulink-PS Converter/RConn1 -- aerodynamic forces/LConn1
  aerodynamic forces/LConn4 -- Simulink-PS Converter3/RConn1
  Simulink-PS Converter5/RConn1 -- aerodynamic forces/LConn6
  Simulink-PS Converter1/RConn1 -- aerodynamic forces/LConn2
  Simulink-PS Converter4/RConn1 -- aerodynamic forces/LConn5
  Blade/LConn1 -- aerodynamic forces/RConn1 -- Weld Joint/RConn1
  240 deg/RConn1 -- Precone/LConn1
  Rhub/RConn1 -- Weld Joint/LConn1
  Rhub/LConn1 -- Precone/RConn1
  Blade1 Root/RConn1 -- 240 deg/LConn1

== system MOST_Lib/Wind turbine/Generator Joint ==
  Gen Torque : Inport
  Generator Joint : sm_lib/Joints/Revolute Joint  JointMode=Normal  CompositeWrenchDir=FollowerOnBase  CompositeWrenchFrame=BaseFrame  SenseConstraintForce=off  SenseConstraintTorque=off  SenseTotalForce=off  SenseTotalTorque=off  PositionTargetSpecify=off  PositionTargetPriority=High  PositionTargetValue=0  PositionTargetValueUnits=deg  VelocityTargetSpecify=on  VelocityTargetPriority=Low  VelocityTargetValue=windTurbine.omega0  VelocityTargetValueUnits=rad/s  EquilibriumPosition=0  EquilibriumPositionUnits=deg  SpringStiffness=0  SpringStiffnessUnits=N*m/deg  DampingCoefficient=0.001  DampingCoefficientUnits=N*m/(deg/s)  LowerLimitSpecify=off  LowerLimitBound=-90  LowerLimitBoundUnits=deg  LowerLimitStiffness=1e4  LowerLimitStiffnessUnits=N*m/deg  LowerLimitDamping=10  LowerLimitDampingUnits=N*m/(deg/s)  LowerLimitTransitionRegionWidth=0.1  LowerLimitTransitionRegionWidthUnits=deg  UpperLimitSpecify=off  UpperLimitBound=90  UpperLimitBoundUnits=deg  UpperLimitStiffness=1e4  UpperLimitStiffnessUnits=N*m/deg  UpperLimitDamping=10  UpperLimitDampingUnits=N*m/(deg/s)  UpperLimitTransitionRegionWidth=0.1  UpperLimitTransitionRegionWidthUnits=deg  TorqueActuationMode=InputTorque  MotionActuationMode=ComputedMotion  SensePosition=on  SenseVelocity=on  SenseAcceleration=off  SenseTorqueForce=off  SenseLowerLimitTorqueForce=off  SenseUpperLimitTorqueForce=off
  PS-Simulink Converter1 : nesl_utility/PS-Simulink Converter  PhysicalDomain=network_engine_domain  SubClassName=ps_output  LeftPortType=input  RightPortType=output  PseudoPeriodic=off  Frequencies=[]  VectorFormat=1-D array  Unit=rad  AffineConversion=off
  PS-Simulink Converter2 : nesl_utility/PS-Simulink Converter  PhysicalDomain=network_engine_domain  SubClassName=ps_output  LeftPortType=input  RightPortType=output  PseudoPeriodic=off  Frequencies=[]  VectorFormat=1-D array  Unit=rad/s  AffineConversion=off
  Rigid Transform4 : sm_lib/Frames and Transforms/Rigid Transform  RotationMethod=StandardAxis  FollAlignAxisA=+X  BaseAlignAxisA=+Y  FollAlignAxisB=+Y  BaseAlignAxisB=+Z  RotationStandardAxis=+Y  RotationAngle=90  RotationAngleUnits=deg  RotationArbitraryAxis=[0 0 1]  RotationSequenceAxes=FollowerAxes  RotationSequence=XYX  RotationSequenceAngles=[0 0 0]  RotationSequenceAnglesUnits=deg  RotationMatrix=[1 0 0; 0 1 0; 0 0 1]  Quaternion=[1 0 0 0]  TranslationMethod=None  TranslationCartesianOffset=[0 0 0]  TranslationCartesianOffsetUnits=m  TranslationStandardAxis=+Z  TranslationStandardOffset=0  TranslationStandardOffsetUnits=m  TranslationROffset=0  TranslationROffsetUnits=m  TranslationThetaOffset=0  TranslationThetaOffsetUnits=deg  TranslationZOffset=0  TranslationZOffsetUnits=m
  Rigid Transform5 : sm_lib/Frames and Transforms/Rigid Transform  RotationMethod=StandardAxis  FollAlignAxisA=+X  BaseAlignAxisA=+Y  FollAlignAxisB=+Y  BaseAlignAxisB=+Z  RotationStandardAxis=-Y  RotationAngle=90  RotationAngleUnits=deg  RotationArbitraryAxis=[0 0 1]  RotationSequenceAxes=FollowerAxes  RotationSequence=XYX  RotationSequenceAngles=[0 0 0]  RotationSequenceAnglesUnits=deg  RotationMatrix=[1 0 0; 0 1 0; 0 0 1]  Quaternion=[1 0 0 0]  TranslationMethod=None  TranslationCartesianOffset=[0 0 0]  TranslationCartesianOffsetUnits=m  TranslationStandardAxis=+Z  TranslationStandardOffset=0  TranslationStandardOffsetUnits=m  TranslationROffset=0  TranslationROffsetUnits=m  TranslationThetaOffset=0  TranslationThetaOffsetUnits=deg  TranslationZOffset=0  TranslationZOffsetUnits=m
  Simulink-PS Converter1 : nesl_utility/Simulink-PS Converter  PhysicalDomain=network_engine_domain  SubClassName=ps_input  LeftPortType=input  RightPortType=output  PseudoPeriodic=off  Frequencies=[]  NoiseDistribution=none  NoiseParameters=[]  Unit=N*m  AffineConversion=off  FilteringAndDerivatives=provide  SimscapeFilterOrder=2  InputFilterTimeConstant=0.1  UdotUserProvided=0
  Conn1 : PMIOPort  Side=Left
  Conn2 : PMIOPort  Port=2  Side=Right
  Azimuth : Outport
  " Rotor speed" : Outport  Port=2
  wires:
  Gen Torque/1 -> Simulink-PS Converter1/1
  PS-Simulink Converter2/1 -> " Rotor speed"/1
  PS-Simulink Converter1/1 -> Azimuth/1
  connections:
  Rigid Transform4/LConn1 -- Conn1/RConn1
  Rigid Transform4/RConn1 -- Generator Joint/LConn1
  PS-Simulink Converter1/LConn1 -- Generator Joint/RConn2
  Simulink-PS Converter1/RConn1 -- Generator Joint/LConn2
  PS-Simulink Converter2/LConn1 -- Generator Joint/RConn3
  Rigid Transform5/RConn1 -- Conn2/RConn1
  Generator Joint/RConn1 -- Rigid Transform5/LConn1

== system MOST_Lib/Wind turbine/Hub ==
  Body Properties Hub : sm_lib/Body Elements/File Solid  ExtGeomFileName=geometry/NREL5MW_Hub.STL  UnitType=Custom  ExtGeomFileUnits=m  StepReaderType=HEX  ExportConvexHullGeometry=off  InertiaType=Custom  BasedOnType=Density  Density=1000  DensityUnits=kg/(m^3)  Mass=windTurbine.hub.mass  MassUnits=kg  CenterOfMass=[0 0 0]  CenterOfMassUnits=m  MomentsOfInertia=windTurbine.hub.inertia  MomentsOfInertiaUnits=kg*m^2  ProductsOfInertia=windTurbine.hub.inertiaProducts  ProductsOfInertiaUnits=kg*m^2  GraphicType=FromGeometry  MarkerShape=Sphere  MarkerSize=10  GraphicVisPropType=AdvancedVisualProperties  GraphicDiffuseColor=[1 1 1]  GraphicOpacity=1  GraphicSpecularColor=[0.5 0.5 0.5 1.0]  GraphicAmbientColor=[0.15 0.15 0.15 1.0]  GraphicEmissiveColor=[0.0 0.0 0.0 1.0]  GraphicShininess=75  DoExposeReferenceFrame=on  SerializedFrames=<Frames/>
  Constant : Constant  Value=-windTurbine.hub.mass*simu.gravity
  External Force and Torque : sm_lib/Forces and Torques/External Force and Torque  EnableForceX=off  EnableForceY=off  EnableForceZ=on  EnableForce=off  ForceResolutionFrame=World  EnableTorqueX=off  EnableTorqueY=off  EnableTorqueZ=off  EnableTorque=off  TorqueResolutionFrame=AttachedFrame
  Simulink-PS Converter : nesl_utility/Simulink-PS Converter  PhysicalDomain=network_engine_domain  SubClassName=ps_input  LeftPortType=input  RightPortType=output  PseudoPeriodic=off  Frequencies=[]  NoiseDistribution=none  NoiseParameters=[]  Unit=1  AffineConversion=off  FilteringAndDerivatives=provide  SimscapeFilterOrder=1  InputFilterTimeConstant=0.001  UdotUserProvided=0
  Hub : PMIOPort  Side=Left
  wires:
  Constant/1 -> Simulink-PS Converter/1
  connections:
  External Force and Torque/RConn1 -- Body Properties Hub/RConn1 -- Hub/RConn1
  Simulink-PS Converter/RConn1 -- External Force and Torque/LConn1

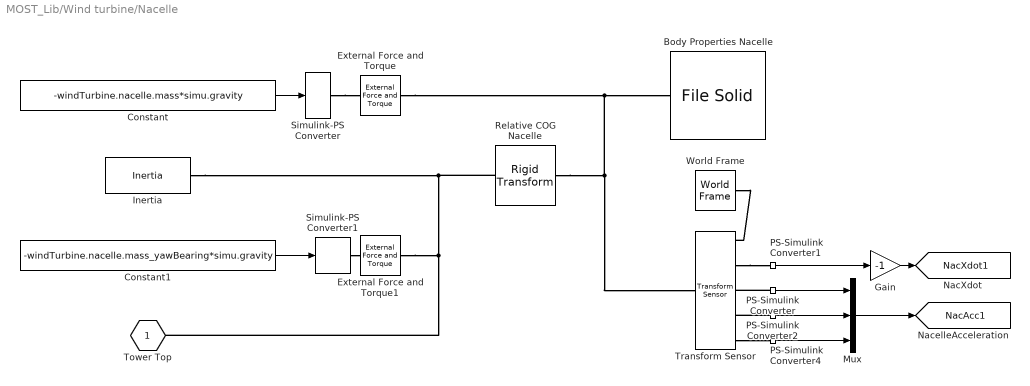
== system MOST_Lib/Wind turbine/Nacelle ==
  Body Properties Nacelle : sm_lib/Body Elements/File Solid  ExtGeomFileName=geometry/NREL5MW_Nacelle.STL  UnitType=Custom  ExtGeomFileUnits=m  StepReaderType=HEX  ExportConvexHullGeometry=off  InertiaType=Custom  BasedOnType=Density  Density=1000  DensityUnits=kg/(m^3)  Mass=windTurbine.nacelle.mass  MassUnits=kg  CenterOfMass=[0 0 0]  CenterOfMassUnits=m  MomentsOfInertia=windTurbine.nacelle.inertia  MomentsOfInertiaUnits=kg*m^2  ProductsOfInertia=windTurbine.nacelle.inertiaProducts  ProductsOfInertiaUnits=kg*m^2  GraphicType=FromGeometry  MarkerShape=Sphere  MarkerSize=10  GraphicVisPropType=SimpleVisualProperties  GraphicDiffuseColor=[1 1 1]  GraphicOpacity=1  GraphicSpecularColor=[0.5 0.5 0.5 1.0]  GraphicAmbientColor=[0.15 0.15 0.15 1.0]  GraphicEmissiveColor=[0.0 0.0 0.0 1.0]  GraphicShininess=75  DoExposeReferenceFrame=on  SerializedFrames=<Frames/>
  Constant : Constant  Value=-windTurbine.nacelle.mass*simu.gravity
  Constant1 : Constant  Value=-windTurbine.nacelle.mass_yawBearing*simu.gravity
  External Force and Torque : sm_lib/Forces and Torques/External Force and Torque  EnableForceX=off  EnableForceY=off  EnableForceZ=on  EnableForce=off  ForceResolutionFrame=World  EnableTorqueX=off  EnableTorqueY=off  EnableTorqueZ=off  EnableTorque=off  TorqueResolutionFrame=AttachedFrame
  External Force and Torque1 : sm_lib/Forces and Torques/External Force and Torque  EnableForceX=off  EnableForceY=off  EnableForceZ=on  EnableForce=off  ForceResolutionFrame=World  EnableTorqueX=off  EnableTorqueY=off  EnableTorqueZ=off  EnableTorque=off  TorqueResolutionFrame=AttachedFrame
  Gain : Gain  Gain=-1
  Inertia : sm_lib/Body Elements/Inertia  InertiaType=PointMass  Mass=windTurbine.nacelle.mass_yawBearing  MassUnits=kg  CenterOfMass=[0 0 0]  CenterOfMassUnits=m  MomentsOfInertia=[1 1 1]  MomentsOfInertiaUnits=kg*m^2  ProductsOfInertia=[0 0 0]  ProductsOfInertiaUnits=kg*m^2  GraphicType=None  MarkerShape=Frame  MarkerSize=20  GraphicVisPropType=SimpleVisualProperties  GraphicDiffuseColor=[0.5 0.5 0.5]  GraphicOpacity=1.0  GraphicSpecularColor=[0.5 0.5 0.5 1.0]  GraphicAmbientColor=[0.15 0.15 0.15 1.0]  GraphicEmissiveColor=[0.0 0.0 0.0 1.0]  GraphicShininess=75
  Mux : Mux  Inputs=3
  PS-Simulink Converter{,1..2,4} (4 alike) : nesl_utility/PS-Simulink Converter  PhysicalDomain=network_engine_domain  SubClassName=ps_output  LeftPortType=input  RightPortType=output  PseudoPeriodic=off  Frequencies=[]  VectorFormat=1-D array  Unit=inherit  AffineConversion=off
  Relative COG Nacelle : sm_lib/Frames and Transforms/Rigid Transform  RotationMethod=None  FollAlignAxisA=+X  BaseAlignAxisA=+Y  FollAlignAxisB=+Y  BaseAlignAxisB=+Z  RotationStandardAxis=+Y  RotationAngle=0.05  RotationAngleUnits=rad  RotationArbitraryAxis=[0.57735026918962584 0.57735026918962584 0.57735026918962584]  RotationSequenceAxes=FollowerAxes  RotationSequence=XYX  RotationSequenceAngles=[0 0 0]  RotationSequenceAnglesUnits=deg  RotationMatrix=[1 0 0; 0 1 0; 0 0 1]  Quaternion=[1 0 0 0]  TranslationMethod=Cartesian  TranslationCartesianOffset=windTurbine.nacelle.cog_rel  TranslationCartesianOffsetUnits=m  TranslationStandardAxis=+Z  TranslationStandardOffset=0  TranslationStandardOffsetUnits=m  TranslationROffset=0  TranslationROffsetUnits=m  TranslationThetaOffset=0  TranslationThetaOffsetUnits=deg  TranslationZOffset=0  TranslationZOffsetUnits=m
  Simulink-PS Converter : nesl_utility/Simulink-PS Converter  PhysicalDomain=network_engine_domain  SubClassName=ps_input  LeftPortType=input  RightPortType=output  PseudoPeriodic=off  Frequencies=[]  NoiseDistribution=none  NoiseParameters=[]  Unit=1  AffineConversion=off  FilteringAndDerivatives=provide  SimscapeFilterOrder=1  InputFilterTimeConstant=0.001  UdotUserProvided=0
  Simulink-PS Converter1 : nesl_utility/Simulink-PS Converter  PhysicalDomain=network_engine_domain  SubClassName=ps_input  LeftPortType=input  RightPortType=output  PseudoPeriodic=off  Frequencies=[]  NoiseDistribution=none  NoiseParameters=[]  Unit=1  AffineConversion=off  FilteringAndDerivatives=provide  SimscapeFilterOrder=1  InputFilterTimeConstant=0.001  UdotUserProvided=0
  Transform Sensor : sm_lib/Frames and Transforms/Transform Sensor  MeasurementFrame=World  RotationSequence=XYX  SenseAngle=off  SenseAxis=off  SenseQ=off  SenseR=off  SenseRotationSequence=off  SenseOmegaX=off  SenseOmegaY=off  SenseOmegaZ=off  SenseOmega=off  SenseQDot=off  SenseRDot=off  SenseRotationSequenceDot=off  SenseAlphaX=off  SenseAlphaY=off  SenseAlphaZ=off  SenseAlpha=off  SenseQDDot=off  SenseRDDot=off  SenseX=off  SenseY=off  SenseZ=off  SenseXYZ=off  SenseRad=off  SenseAzim=off  SenseDist=off  SenseInc=off  SenseXDot=on  SenseYDot=off  SenseZDot=off  SenseXYZDot=off  SenseRadDot=off  SenseAzimDot=off  SenseDistDot=off  SenseIncDot=off  SenseXDDot=on  SenseYDDot=on  SenseZDDot=on  SenseXYZDDot=off  SenseRadDDot=off  SenseAzimDDot=off  SenseDistDDot=off  SenseIncDDot=off
  World Frame : sm_lib/Frames and Transforms/World Frame
  Tower Top : PMIOPort  Side=Left
  tag scope: NacAcc1=global, NacXdot1=global
  wires:
  Constant/1 -> Simulink-PS Converter/1
  Constant1/1 -> Simulink-PS Converter1/1
  PS-Simulink Converter4/1 -> Mux/3
  PS-Simulink Converter2/1 -> Mux/2
  PS-Simulink Converter1/1 -> Gain/1
  PS-Simulink Converter/1 -> Mux/1
  Gain/1 -> [NacXdot1]
  Mux/1 -> [NacAcc1]
  connections:
  Inertia/RConn1 -- Relative COG Nacelle/LConn1 -- External Force and Torque1/RConn1 -- Tower Top/RConn1
  Simulink-PS Converter/RConn1 -- External Force and Torque/LConn1
  Simulink-PS Converter1/RConn1 -- External Force and Torque1/LConn1
  PS-Simulink Converter2/LConn1 -- Transform Sensor/RConn4
  Transform Sensor/RConn2 -- PS-Simulink Converter1/LConn1
  World Frame/RConn1 -- Transform Sensor/RConn1
  Relative COG Nacelle/RConn1 -- Transform Sensor/LConn1 -- Body Properties Nacelle/RConn1 -- External Force and Torque/RConn1
  Transform Sensor/RConn5 -- PS-Simulink Converter4/LConn1
  PS-Simulink Converter/LConn1 -- Transform Sensor/RConn3

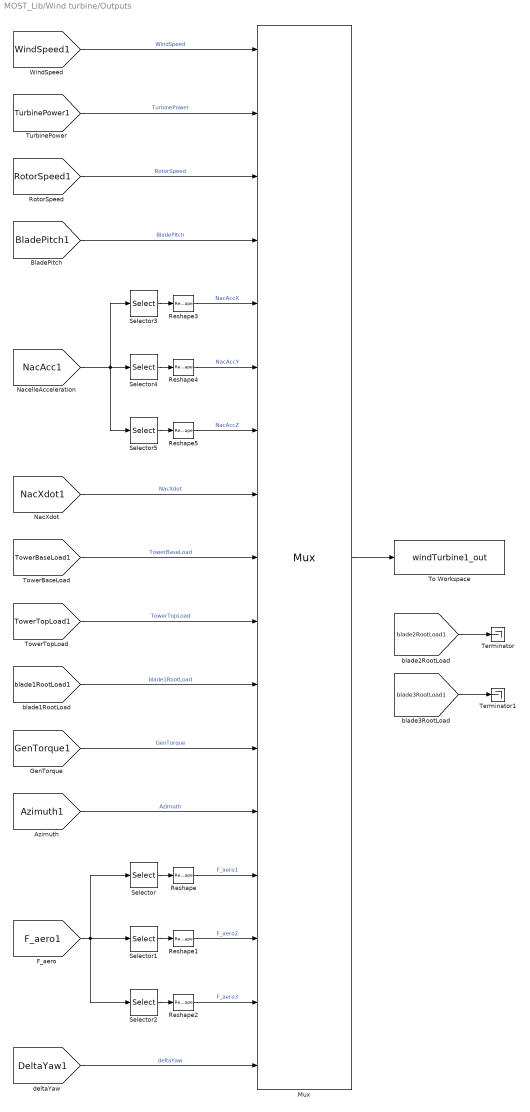
== system MOST_Lib/Wind turbine/Outputs ==
  Mux : Mux  Inputs=17
      settings: DisplayOption=signals
  Reshape{,1..5} (6 alike) : Reshape
  Selector : Selector  NumberOfDimensions=2  InputPortWidth=3  IndexOptions=Select all,Index vector (dialog)  Indices=[1 3],1  OutputSizes=1,1
  Selector1 : Selector  NumberOfDimensions=2  InputPortWidth=3  IndexOptions=Select all,Index vector (dialog)  Indices=[1 3],2  OutputSizes=1,1
  Selector2 : Selector  NumberOfDimensions=2  InputPortWidth=3  IndexOptions=Select all,Index vector (dialog)  Indices=[1 3],3  OutputSizes=1,1
  Selector3 : Selector  NumberOfDimensions=2  InputPortWidth=3  IndexOptions=Select all,Index vector (dialog)  Indices=[1 3],1  OutputSizes=1,1
  Selector4 : Selector  NumberOfDimensions=2  InputPortWidth=3  IndexOptions=Select all,Index vector (dialog)  Indices=[1 3],2  OutputSizes=1,1
  Selector5 : Selector  NumberOfDimensions=2  InputPortWidth=3  IndexOptions=Select all,Index vector (dialog)  Indices=[1 3],3  OutputSizes=1,1
  Terminator : Terminator
  Terminator1 : Terminator
  To Workspace : ToWorkspace  VariableName=windTurbine1_out  SaveFormat=Structure With Time  SampleTime=simu.dtOut
  wires:
  Mux/1 -> To Workspace/1
  [blade2RootLoad1] -> Terminator/1
  [blade3RootLoad1] -> Terminator1/1
  [BladePitch1] -> Mux/4  "BladePitch"
  [RotorSpeed1] -> Mux/3  "RotorSpeed"
  [TurbinePower1] -> Mux/2  "TurbinePower"
  [NacAcc1] -> Selector3/1, Selector5/1, Selector4/1
  [TowerBaseLoad1] -> Mux/9  "TowerBaseLoad"
  [TowerTopLoad1] -> Mux/10  "TowerTopLoad"
  [blade1RootLoad1] -> Mux/11  "blade1RootLoad"
  [GenTorque1] -> Mux/12  "GenTorque"
  [Azimuth1] -> Mux/13  "Azimuth"
  [WindSpeed1] -> Mux/1  "WindSpeed"
  [F_aero1] -> Selector/1, Selector2/1, Selector1/1
  Selector/1 -> Reshape/1
  Selector1/1 -> Reshape1/1
  Selector2/1 -> Reshape2/1
  Reshape/1 -> Mux/14  "F_aero1"
  Reshape1/1 -> Mux/15  "F_aero2"
  Reshape2/1 -> Mux/16  "F_aero3"
  [DeltaYaw1] -> Mux/17  "deltaYaw"
  Selector4/1 -> Reshape4/1
  Selector3/1 -> Reshape3/1
  Selector5/1 -> Reshape5/1
  Reshape3/1 -> Mux/5  "NacAccX"
  Reshape4/1 -> Mux/6  "NacAccY"
  Reshape5/1 -> Mux/7  "NacAccZ"
  [NacXdot1] -> Mux/8  "NacXdot"
